simulink model "V2x_TC_CarBreakdownWarning_cs"  (Simulink 7.6)
settings: Solver=ode5  SolverMode=SingleTasking  StartTime=0.0  StopTime=18  FixedStep=1/100  RelTol=1e-3
PreLoadFcn:
  | check_NUTS_defined;
  | 
  | assignin('base',['model_closed_' bdroot],false);addpath('../includes_V2x');
InitFcn:
  | PreScanExperimentInitFcn(bdroot)
StopFcn:
  | PreScanExperimentStopFcn(bdroot)
undefined symbols (not defined in the file or in its folder): acceleration, actorID, actorType, DiscIntNeverNeededParam, GPS_alt, GPS_lat, GPS_long, intmax, lightBarInUse, messageID, Newton, publicActorType, Raphson, rotZ, sigbuilder_block, sireneInUse, trafficLightPriority, turnAdvice, velocity, x_ini_VRML, y_ini_VRML, yawRate, z_ini_VRML
libraries: simulink x61, PreScanSimulinkLibrary x19, PreScanUsefulBlocks x7, simulink_extras x1
(part 5 of 10)

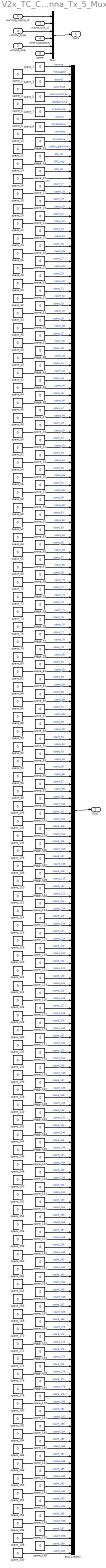
== system V2x_TC_CarBreakdownWarning_cs/BMW_X5_1/Antenna_Tx_5_Mux ==
  warning_signal_id : Inport  SampleTime=TimeStep
  maneuvre_id : Inport  Port=2  SampleTime=TimeStep
  vehicle_type : Inport  Port=3  SampleTime=TimeStep
  brakingcapacity : Inport  Port=4  SampleTime=TimeStep
  vehicle_size : Inport  Port=5  SampleTime=TimeStep
  spare : Inport  Port=6  SampleTime=TimeStep
  Bus Creator : BusCreator  Inputs=200
  Mux : Mux  Inputs=6
  spare_{1..200} (200 alike) : Constant  Value=0  SampleTime=TimeStep
  Out1 : Outport
  Out2 : Outport  Port=2  SampleTime=TimeStep
  wires:
  spare_200/1 -> Bus Creator/200  "spare_200"
  spare_199/1 -> Bus Creator/199  "spare_199"
  spare_198/1 -> Bus Creator/198  "spare_198"
  spare_197/1 -> Bus Creator/197  "spare_197"
  spare_196/1 -> Bus Creator/196  "spare_196"
  spare_195/1 -> Bus Creator/195  "spare_195"
  spare_194/1 -> Bus Creator/194  "spare_194"
  spare_193/1 -> Bus Creator/193  "spare_193"
  spare_192/1 -> Bus Creator/192  "spare_192"
  spare_191/1 -> Bus Creator/191  "spare_191"
  spare_190/1 -> Bus Creator/190  "spare_190"
  spare_189/1 -> Bus Creator/189  "spare_189"
  spare_188/1 -> Bus Creator/188  "spare_188"
  spare_187/1 -> Bus Creator/187  "spare_187"
  spare_186/1 -> Bus Creator/186  "spare_186"
  spare_185/1 -> Bus Creator/185  "spare_185"
  spare_184/1 -> Bus Creator/184  "spare_184"
  spare_183/1 -> Bus Creator/183  "spare_183"
  spare_182/1 -> Bus Creator/182  "spare_182"
  spare_181/1 -> Bus Creator/181  "spare_181"
  spare_180/1 -> Bus Creator/180  "spare_180"
  spare_179/1 -> Bus Creator/179  "spare_179"
  spare_178/1 -> Bus Creator/178  "spare_178"
  spare_177/1 -> Bus Creator/177  "spare_177"
  spare_176/1 -> Bus Creator/176  "spare_176"
  spare_175/1 -> Bus Creator/175  "spare_175"
  spare_174/1 -> Bus Creator/174  "spare_174"
  spare_173/1 -> Bus Creator/173  "spare_173"
  spare_172/1 -> Bus Creator/172  "spare_172"
  spare_171/1 -> Bus Creator/171  "spare_171"
  spare_170/1 -> Bus Creator/170  "spare_170"
  spare_169/1 -> Bus Creator/169  "spare_169"
  spare_168/1 -> Bus Creator/168  "spare_168"
  spare_167/1 -> Bus Creator/167  "spare_167"
  spare_166/1 -> Bus Creator/166  "spare_166"
  spare_165/1 -> Bus Creator/165  "spare_165"
  spare_164/1 -> Bus Creator/164  "spare_164"
  spare_163/1 -> Bus Creator/163  "spare_163"
  spare_162/1 -> Bus Creator/162  "spare_162"
  spare_161/1 -> Bus Creator/161  "spare_161"
  spare_160/1 -> Bus Creator/160  "spare_160"
  spare_159/1 -> Bus Creator/159  "spare_159"
  spare_158/1 -> Bus Creator/158  "spare_158"
  spare_157/1 -> Bus Creator/157  "spare_157"
  spare_156/1 -> Bus Creator/156  "spare_156"
  spare_155/1 -> Bus Creator/155  "spare_155"
  spare_154/1 -> Bus Creator/154  "spare_154"
  spare_153/1 -> Bus Creator/153  "spare_153"
  spare_152/1 -> Bus Creator/152  "spare_152"
  spare_151/1 -> Bus Creator/151  "spare_151"
  spare_150/1 -> Bus Creator/150  "spare_150"
  spare_149/1 -> Bus Creator/149  "spare_149"
  spare_148/1 -> Bus Creator/148  "spare_148"
  spare_147/1 -> Bus Creator/147  "spare_147"
  spare_146/1 -> Bus Creator/146  "spare_146"
  spare_145/1 -> Bus Creator/145  "spare_145"
  spare_144/1 -> Bus Creator/144  "spare_144"
  spare_143/1 -> Bus Creator/143  "spare_143"
  spare_142/1 -> Bus Creator/142  "spare_142"
  spare_141/1 -> Bus Creator/141  "spare_141"
  spare_140/1 -> Bus Creator/140  "spare_140"
  spare_139/1 -> Bus Creator/139  "spare_139"
  spare_138/1 -> Bus Creator/138  "spare_138"
  spare_137/1 -> Bus Creator/137  "spare_137"
  spare_136/1 -> Bus Creator/136  "spare_136"
  spare_135/1 -> Bus Creator/135  "spare_135"
  spare_134/1 -> Bus Creator/134  "spare_134"
  spare_133/1 -> Bus Creator/133  "spare_133"
  spare_132/1 -> Bus Creator/132  "spare_132"
  spare_131/1 -> Bus Creator/131  "spare_131"
  spare_130/1 -> Bus Creator/130  "spare_130"
  spare_129/1 -> Bus Creator/129  "spare_129"
  spare_128/1 -> Bus Creator/128  "spare_128"
  spare_127/1 -> Bus Creator/127  "spare_127"
  spare_126/1 -> Bus Creator/126  "spare_126"
  spare_125/1 -> Bus Creator/125  "spare_125"
  spare_124/1 -> Bus Creator/124  "spare_124"
  spare_123/1 -> Bus Creator/123  "spare_123"
  spare_122/1 -> Bus Creator/122  "spare_122"
  spare_121/1 -> Bus Creator/121  "spare_121"
  spare_120/1 -> Bus Creator/120  "spare_120"
  spare_119/1 -> Bus Creator/119  "spare_119"
  spare_118/1 -> Bus Creator/118  "spare_118"
  spare_117/1 -> Bus Creator/117  "spare_117"
  spare_116/1 -> Bus Creator/116  "spare_116"
  spare_115/1 -> Bus Creator/115  "spare_115"
  spare_114/1 -> Bus Creator/114  "spare_114"
  spare_113/1 -> Bus Creator/113  "spare_113"
  spare_112/1 -> Bus Creator/112  "spare_112"
  spare_111/1 -> Bus Creator/111  "spare_111"
  spare_110/1 -> Bus Creator/110  "spare_110"
  spare_109/1 -> Bus Creator/109  "spare_109"
  spare_108/1 -> Bus Creator/108  "spare_108"
  spare_107/1 -> Bus Creator/107  "spare_107"
  spare_106/1 -> Bus Creator/106  "spare_106"
  spare_105/1 -> Bus Creator/105  "spare_105"
  spare_104/1 -> Bus Creator/104  "spare_104"
  spare_103/1 -> Bus Creator/103  "spare_103"
  spare_102/1 -> Bus Creator/102  "spare_102"
  spare_101/1 -> Bus Creator/101  "spare_101"
  spare_100/1 -> Bus Creator/100  "spare_100"
  spare_99/1 -> Bus Creator/99  "spare_99"
  spare_98/1 -> Bus Creator/98  "spare_98"
  spare_97/1 -> Bus Creator/97  "spare_97"
  spare_96/1 -> Bus Creator/96  "spare_96"
  spare_95/1 -> Bus Creator/95  "spare_95"
  spare_94/1 -> Bus Creator/94  "spare_94"
  spare_93/1 -> Bus Creator/93  "spare_93"
  spare_92/1 -> Bus Creator/92  "spare_92"
  spare_91/1 -> Bus Creator/91  "spare_91"
  spare_90/1 -> Bus Creator/90  "spare_90"
  spare_89/1 -> Bus Creator/89  "spare_89"
  spare_88/1 -> Bus Creator/88  "spare_88"
  spare_87/1 -> Bus Creator/87  "spare_87"
  spare_86/1 -> Bus Creator/86  "spare_86"
  spare_85/1 -> Bus Creator/85  "spare_85"
  spare_84/1 -> Bus Creator/84  "spare_84"
  spare_83/1 -> Bus Creator/83  "spare_83"
  spare_82/1 -> Bus Creator/82  "spare_82"
  spare_81/1 -> Bus Creator/81  "spare_81"
  spare_80/1 -> Bus Creator/80  "spare_80"
  spare_79/1 -> Bus Creator/79  "spare_79"
  spare_78/1 -> Bus Creator/78  "spare_78"
  spare_77/1 -> Bus Creator/77  "spare_77"
  spare_76/1 -> Bus Creator/76  "spare_76"
  spare_75/1 -> Bus Creator/75  "spare_75"
  spare_74/1 -> Bus Creator/74  "spare_74"
  spare_73/1 -> Bus Creator/73  "spare_73"
  spare_72/1 -> Bus Creator/72  "spare_72"
  spare_71/1 -> Bus Creator/71  "spare_71"
  spare_70/1 -> Bus Creator/70  "spare_70"
  spare_69/1 -> Bus Creator/69  "spare_69"
  spare_68/1 -> Bus Creator/68  "spare_68"
  spare_67/1 -> Bus Creator/67  "spare_67"
  spare_66/1 -> Bus Creator/66  "spare_66"
  spare_65/1 -> Bus Creator/65  "spare_65"
  spare_64/1 -> Bus Creator/64  "spare_64"
  spare_63/1 -> Bus Creator/63  "spare_63"
  spare_62/1 -> Bus Creator/62  "spare_62"
  spare_61/1 -> Bus Creator/61  "spare_61"
  spare_60/1 -> Bus Creator/60  "spare_60"
  spare_59/1 -> Bus Creator/59  "spare_59"
  spare_58/1 -> Bus Creator/58  "spare_58"
  spare_57/1 -> Bus Creator/57  "spare_57"
  spare_56/1 -> Bus Creator/56  "spare_56"
  spare_55/1 -> Bus Creator/55  "spare_55"
  spare_54/1 -> Bus Creator/54  "spare_54"
  spare_53/1 -> Bus Creator/53  "spare_53"
  spare_52/1 -> Bus Creator/52  "spare_52"
  spare_51/1 -> Bus Creator/51  "spare_51"
  spare_50/1 -> Bus Creator/50  "spare_50"
  spare_49/1 -> Bus Creator/49  "spare_49"
  spare_48/1 -> Bus Creator/48  "spare_48"
  spare_47/1 -> Bus Creator/47  "spare_47"
  spare_46/1 -> Bus Creator/46  "spare_46"
  spare_45/1 -> Bus Creator/45  "spare_45"
  spare_44/1 -> Bus Creator/44  "spare_44"
  spare_43/1 -> Bus Creator/43  "spare_43"
  spare_42/1 -> Bus Creator/42  "spare_42"
  spare_41/1 -> Bus Creator/41  "spare_41"
  spare_40/1 -> Bus Creator/40  "spare_40"
  spare_39/1 -> Bus Creator/39  "spare_39"
  spare_38/1 -> Bus Creator/38  "spare_38"
  spare_37/1 -> Bus Creator/37  "spare_37"
  spare_36/1 -> Bus Creator/36  "spare_36"
  spare_35/1 -> Bus Creator/35  "spare_35"
  spare_34/1 -> Bus Creator/34  "spare_34"
  spare_33/1 -> Bus Creator/33  "spare_33"
  spare_32/1 -> Bus Creator/32  "spare_32"
  spare_31/1 -> Bus Creator/31  "spare_31"
  spare_30/1 -> Bus Creator/30  "spare_30"
  spare_29/1 -> Bus Creator/29  "spare_29"
  spare_28/1 -> Bus Creator/28  "spare_28"
  spare_27/1 -> Bus Creator/27  "spare_27"
  spare_26/1 -> Bus Creator/26  "spare_26"
  spare_25/1 -> Bus Creator/25  "spare_25"
  spare_24/1 -> Bus Creator/24  "spare_24"
  spare_23/1 -> Bus Creator/23  "spare_23"
  spare_22/1 -> Bus Creator/22  "spare_22"
  spare_21/1 -> Bus Creator/21  "spare_21"
  spare_19/1 -> Bus Creator/19  "spare_19"
  spare_18/1 -> Bus Creator/18  "spare_18"
  spare_17/1 -> Bus Creator/17  "spare_17"
  warning_signal_id/1 -> Mux/1
  maneuvre_id/1 -> Mux/2
  vehicle_type/1 -> Mux/3
  brakingcapacity/1 -> Mux/4
  vehicle_size/1 -> Mux/5
  Mux/1 -> Out1/1
  Bus Creator/1 -> Out2/1
  spare/1 -> Mux/6
  spare_1/1 -> Bus Creator/1  "warning"
  spare_2/1 -> Bus Creator/2  "messageID"
  spare_3/1 -> Bus Creator/3  "actorID"
  spare_4/1 -> Bus Creator/4  "actorType"
  spare_5/1 -> Bus Creator/5  "publicActorType"
  spare_6/1 -> Bus Creator/6  "lightBarInUse"
  spare_7/1 -> Bus Creator/7  "sireneInUse"
  spare_8/1 -> Bus Creator/8  "velocity"
  spare_9/1 -> Bus Creator/9  "acceleration"
  spare_10/1 -> Bus Creator/10  "yawRate"
  spare_11/1 -> Bus Creator/11  "turnAdvice"
  spare_12/1 -> Bus Creator/12  "trafficLightPriority"
  spare_13/1 -> Bus Creator/13  "GPS_lat"
  spare_14/1 -> Bus Creator/14  "GPS_long"
  spare_15/1 -> Bus Creator/15  "GPS_alt"
  spare_16/1 -> Bus Creator/16  "rotZ"
  spare_20/1 -> Bus Creator/20  "spare_20"

== system V2x_TC_CarBreakdownWarning_cs/BMW_X5_1/SELF_Demux ==
  SELF : Inport
  Demux1 : Demux  Outputs=3
  Demux2 : Demux  Outputs=3
  Demux3 : Demux  Outputs=[3 3 1 1]
  Demux4 : Demux  Outputs=3
  Gain : Gain  Gain=180/pi
  Gain1 : Gain  Gain=180/pi
  Selector : Selector  InputPortWidth=3  IndexOptions=Index vector (dialog)  Indices=[3]  OutputSizes=1
  compas converter : Subsystem
  xyz2GPS : PreScanUsefulBlocks/xyz2GPS  CoordinateCount=1  GPS_base=[0.000000 0.000000 0.000]
  x [m] : Outport
  y [m] : Outport  Port=2
  z [m] : Outport  Port=3
  rotx [deg] : Outport  Port=4
  roty [deg] : Outport  Port=5
  rotz [deg] : Outport  Port=6
  GPS lat [deg] : Outport  Port=7
  GPS long [deg] : Outport  Port=8
  GPS alt [m] : Outport  Port=9
  velocity [m/s] : Outport  Port=10
  heading [deg] : Outport  Port=11
  yaw rate [deg/s] : Outport  Port=12
  wires:
  Demux3/4 -> Gain1/1
  Gain1/1 -> yaw rate [deg/s]/1
  Demux3/3 -> velocity [m/s]/1
  compas converter/1(heading [deg]) -> heading [deg]/1
  xyz2GPS/1 -> Demux4/1
  Demux4/3 -> GPS alt [m]/1
  Demux4/2 -> GPS long [deg]/1
  Demux4/1 -> GPS lat [deg]/1
  Demux3/2 -> Gain/1, Selector/1
  Demux3/1 -> xyz2GPS/1, Demux1/1
  SELF/1 -> Demux3/1
  Demux2/3 -> rotz [deg]/1
  Demux2/2 -> roty [deg]/1
  Demux2/1 -> rotx [deg]/1
  Demux1/3 -> z [m]/1
  Demux1/2 -> y [m]/1
  Demux1/1 -> x [m]/1
  Gain/1 -> Demux2/1
  Selector/1 -> compas converter/1(rotz [rad])

== system V2x_TC_CarBreakdownWarning_cs/BMW_X5_1/Trajectories ==
  Traj2State1 : Subsystem  Tag=Traj2State
      settings: DeleteFcn=PreScanBlockDeleteFcn;
      mask Type: PreScan Demux Block:
  Trajectory_4 : Subsystem  Tag=Trajectory  mask(PreScan Source Block: Trajectory){FileName='Trajectory_4.mat', TimeStep=1/100}
      mask prompts: TimeStep "Time Step [s]"
      mask help:
      | The Trajectory block contains the trajectories defined in the PreScan Experiment Editor. The output of the trajectory block is the (vehicle) State.
      |
      | For more information, please click Help.
      mask init: same as V2x_TC_CarBreakdownWarning_cs/Audi_A8_1/Trajectories/Trajectory_1
      settings: DeleteFcn=PreScanBlockDeleteFcn;
      mask Help: eval('openHelp(312)')
      mask Display: fprintf(FileName)
  Trajectory_4_Offset : Constant  Tag=TrajectoryOffset  Value="[0  0  0  0  0  0]"
  State : Outport  Tag=TrajOutport
  wires:
  Trajectory_4/1(trajectory) -> Traj2State1/1(Traj Org)
  Trajectory_4_Offset/1 -> Traj2State1/2(Offset)
  Traj2State1/1(state) -> State/1

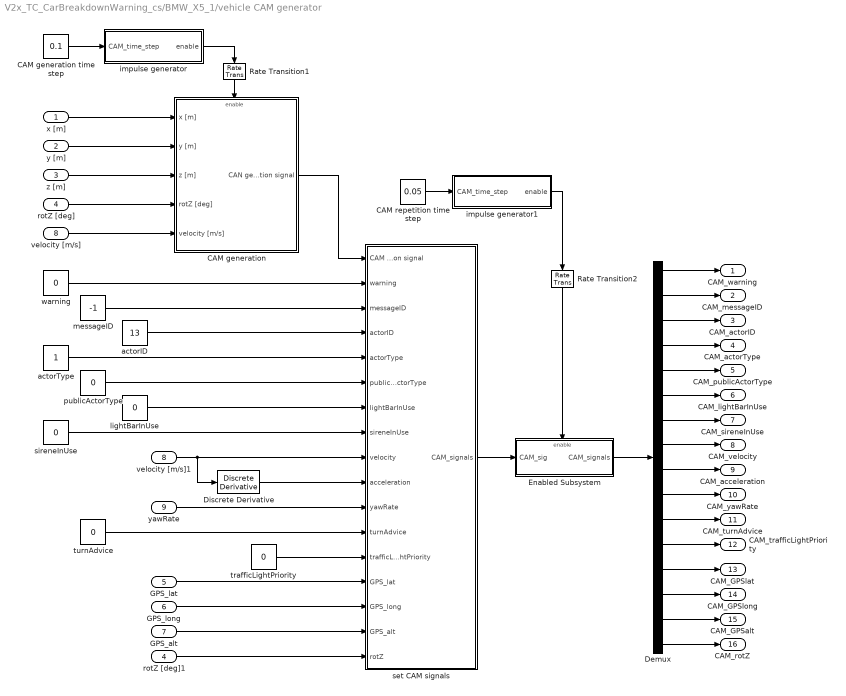
== system V2x_TC_CarBreakdownWarning_cs/BMW_X5_1/vehicle CAM generator ==
  x [m] : Inport
  y [m] : Inport  Port=2
  z [m] : Inport  Port=3
  rotZ [deg] : Inport  Port=4
  GPS_lat : Inport  Port=5
  GPS_long : Inport  Port=6
  GPS_alt : Inport  Port=7
  velocity [m/s] : Inport  Port=8
  yawRate : Inport  Port=9
  CAM generation : Subsystem  TreatAsAtomicUnit=on
  CAM generation time step : Constant  Value=0.1
  CAM repetition time step : Constant  Value=0.05
  Demux : Demux  Outputs=16
  Discrete Derivative : simulink/Discrete/Discrete Derivative  SystemSampleTime=-1  gainval=1.0  ICPrevScaledInput=0.0  OutMin=[]  OutMax=[]  OutDataType=fixdt(1, 16)  OutScaling=2^-10  DoSatur=off
  Enabled Subsystem : Subsystem  TreatAsAtomicUnit=on
  Rate Transition1 : RateTransition  Integrity=off  OutPortSampleTimeOpt=Inherit
  Rate Transition2 : RateTransition  Integrity=off  OutPortSampleTimeOpt=Inherit
  actorID : Constant  Value=13
  actorType : Constant
  impulse generator : Subsystem
  impulse generator1 : Subsystem
  lightBarInUse : Constant  Value=0
  messageID : Constant  Value=-1
  publicActorType : Constant  Value=0
  rotZ [deg]1 : InportShadow  Port=4
  set CAM signals : Subsystem
  sireneInUse : Constant  Value=0
  trafficLightPriority : Constant  Value=0
  turnAdvice : Constant  Value=0
  velocity [m/s]1 : InportShadow  Port=8
  warning : Constant  Value=0
  CAM_warning : Outport
  CAM_messageID : Outport  Port=2
  CAM_actorID : Outport  Port=3
  CAM_actorType : Outport  Port=4
  CAM_publicActorType : Outport  Port=5
  CAM_lightBarInUse : Outport  Port=6
  CAM_sireneInUse : Outport  Port=7
  CAM_velocity : Outport  Port=8
  CAM_acceleration : Outport  Port=9
  CAM_yawRate : Outport  Port=10
  CAM_turnAdvice : Outport  Port=11
  CAM_trafficLightPriority : Outport  Port=12
  CAM_GPSlat : Outport  Port=13
  CAM_GPSlong : Outport  Port=14
  CAM_GPSalt : Outport  Port=15
  CAM_rotZ : Outport  Port=16
  wires:
  CAM generation time step/1 -> impulse generator/1(CAM_time_step)
  CAM repetition time step/1 -> impulse generator1/1(CAM_time_step)
  impulse generator1/1(enable) -> Rate Transition2/1
  warning/1 -> set CAM signals/2(warning)
  messageID/1 -> set CAM signals/3(messageID)
  actorID/1 -> set CAM signals/4(actorID)
  actorType/1 -> set CAM signals/5(actorType)
  publicActorType/1 -> set CAM signals/6(publicActorType)
  lightBarInUse/1 -> set CAM signals/7(lightBarInUse)
  sireneInUse/1 -> set CAM signals/8(sireneInUse)
  velocity [m/s]1/1 -> Discrete Derivative/1, set CAM signals/9(velocity)
  Discrete Derivative/1 -> set CAM signals/10(acceleration)
  yawRate/1 -> set CAM signals/11(yawRate)
  turnAdvice/1 -> set CAM signals/12(turnAdvice)
  trafficLightPriority/1 -> set CAM signals/13(trafficLightPriority)
  GPS_lat/1 -> set CAM signals/14(GPS_lat)
  GPS_long/1 -> set CAM signals/15(GPS_long)
  GPS_alt/1 -> set CAM signals/16(GPS_alt)
  rotZ [deg]1/1 -> set CAM signals/17(rotZ)
  CAM generation/1(CAN generation signal) -> set CAM signals/1(CAM generation signal)
  x [m]/1 -> CAM generation/1(x [m])
  y [m]/1 -> CAM generation/2(y [m])
  z [m]/1 -> CAM generation/3(z [m])
  rotZ [deg]/1 -> CAM generation/4(rotZ [deg])
  velocity [m/s]/1 -> CAM generation/5(velocity [m/s])
  impulse generator/1(enable) -> Rate Transition1/1
  Rate Transition1/1 -> CAM generation/Enable
  set CAM signals/1(CAM_signals) -> Enabled Subsystem/1(CAM_sig)
  Rate Transition2/1 -> Enabled Subsystem/Enable
  Enabled Subsystem/1(CAM_signals) -> Demux/1
  Demux/1 -> CAM_warning/1
  Demux/2 -> CAM_messageID/1
  Demux/3 -> CAM_actorID/1
  Demux/4 -> CAM_actorType/1
  Demux/5 -> CAM_publicActorType/1
  Demux/6 -> CAM_lightBarInUse/1
  Demux/7 -> CAM_sireneInUse/1
  Demux/8 -> CAM_velocity/1
  Demux/9 -> CAM_acceleration/1
  Demux/10 -> CAM_yawRate/1
  Demux/11 -> CAM_turnAdvice/1
  Demux/12 -> CAM_trafficLightPriority/1
  Demux/13 -> CAM_GPSlat/1
  Demux/14 -> CAM_GPSlong/1
  Demux/15 -> CAM_GPSalt/1
  Demux/16 -> CAM_rotZ/1

== system V2x_TC_CarBreakdownWarning_cs/CameraTrolley/Dynamics_Empty ==
  note: For state mode 'Dynamic' positions
      | are not taken into account, as they
      | are computed by integrating velocity.
      | Click annotation for Help.
  Ground_{1..9} (9 alike) : Ground
  MuxState : Subsystem  Tag=MuxState  mask{positioningmode=on, TimeStep=1/100}
      mask prompts: positioningmode "Positioning Mode"; TimeStep "Auto Assigned: Time Step [s]"
      settings: DeleteFcn=PreScanBlockDeleteFcn;
  State : Outport  Tag=StateOutport
  wires:
  MuxState/1(state) -> State/1
  Ground_1/1 -> MuxState/1(x [m])
  Ground_2/1 -> MuxState/2(y [m])
  Ground_3/1 -> MuxState/3(z [m])
  Ground_4/1 -> MuxState/4(dx [m/s])
  Ground_5/1 -> MuxState/5(dy [m/s])
  Ground_6/1 -> MuxState/6(dz [m/s])
  Ground_7/1 -> MuxState/7(R [rad])
  Ground_8/1 -> MuxState/8(P [rad])
  Ground_9/1 -> MuxState/9(Y [rad])

== system V2x_TC_CarBreakdownWarning_cs/CameraTrolley/SELF_Demux ==
  SELF : Inport
  Demux1 : Demux  Outputs=3
  Demux2 : Demux  Outputs=3
  Demux3 : Demux  Outputs=[3 3 1 1]
  Demux4 : Demux  Outputs=3
  Gain : Gain  Gain=180/pi
  Gain1 : Gain  Gain=180/pi
  Selector : Selector  InputPortWidth=3  IndexOptions=Index vector (dialog)  Indices=[3]  OutputSizes=1
  compas converter : Subsystem
  xyz2GPS : PreScanUsefulBlocks/xyz2GPS  CoordinateCount=1  GPS_base=[0.000000 0.000000 0.000]
  x [m] : Outport
  y [m] : Outport  Port=2
  z [m] : Outport  Port=3
  rotx [deg] : Outport  Port=4
  roty [deg] : Outport  Port=5
  rotz [deg] : Outport  Port=6
  GPS lat [deg] : Outport  Port=7
  GPS long [deg] : Outport  Port=8
  GPS alt [m] : Outport  Port=9
  velocity [m/s] : Outport  Port=10
  heading [deg] : Outport  Port=11
  yaw rate [deg/s] : Outport  Port=12
  wires:
  Demux3/4 -> Gain1/1
  Gain1/1 -> yaw rate [deg/s]/1
  Demux3/3 -> velocity [m/s]/1
  compas converter/1(heading [deg]) -> heading [deg]/1
  xyz2GPS/1 -> Demux4/1
  Demux4/3 -> GPS alt [m]/1
  Demux4/2 -> GPS long [deg]/1
  Demux4/1 -> GPS lat [deg]/1
  Demux3/2 -> Gain/1, Selector/1
  Demux3/1 -> xyz2GPS/1, Demux1/1
  SELF/1 -> Demux3/1
  Demux2/3 -> rotz [deg]/1
  Demux2/2 -> roty [deg]/1
  Demux2/1 -> rotx [deg]/1
  Demux1/3 -> z [m]/1
  Demux1/2 -> y [m]/1
  Demux1/1 -> x [m]/1
  Gain/1 -> Demux2/1
  Selector/1 -> compas converter/1(rotz [rad])

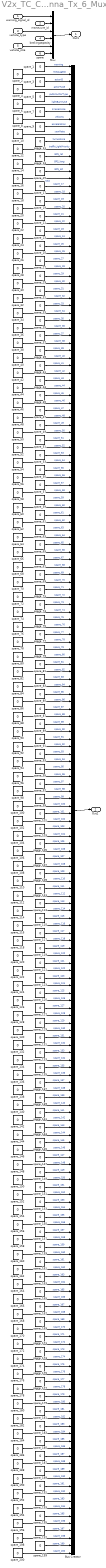
== system V2x_TC_CarBreakdownWarning_cs/Fiat_Bravo_1/Antenna_Tx_6_Mux ==
  warning_signal_id : Inport  SampleTime=TimeStep
  maneuvre_id : Inport  Port=2  SampleTime=TimeStep
  vehicle_type : Inport  Port=3  SampleTime=TimeStep
  brakingcapacity : Inport  Port=4  SampleTime=TimeStep
  vehicle_size : Inport  Port=5  SampleTime=TimeStep
  spare : Inport  Port=6  SampleTime=TimeStep
  Bus Creator : BusCreator  Inputs=200
  Mux : Mux  Inputs=6
  spare_{1..200} (200 alike) : Constant  Value=0  SampleTime=TimeStep
  Out1 : Outport
  Out2 : Outport  Port=2  SampleTime=TimeStep
  wires:
  spare_200/1 -> Bus Creator/200  "spare_200"
  spare_199/1 -> Bus Creator/199  "spare_199"
  spare_198/1 -> Bus Creator/198  "spare_198"
  spare_197/1 -> Bus Creator/197  "spare_197"
  spare_196/1 -> Bus Creator/196  "spare_196"
  spare_195/1 -> Bus Creator/195  "spare_195"
  spare_194/1 -> Bus Creator/194  "spare_194"
  spare_193/1 -> Bus Creator/193  "spare_193"
  spare_192/1 -> Bus Creator/192  "spare_192"
  spare_191/1 -> Bus Creator/191  "spare_191"
  spare_190/1 -> Bus Creator/190  "spare_190"
  spare_189/1 -> Bus Creator/189  "spare_189"
  spare_188/1 -> Bus Creator/188  "spare_188"
  spare_187/1 -> Bus Creator/187  "spare_187"
  spare_186/1 -> Bus Creator/186  "spare_186"
  spare_185/1 -> Bus Creator/185  "spare_185"
  spare_184/1 -> Bus Creator/184  "spare_184"
  spare_183/1 -> Bus Creator/183  "spare_183"
  spare_182/1 -> Bus Creator/182  "spare_182"
  spare_181/1 -> Bus Creator/181  "spare_181"
  spare_180/1 -> Bus Creator/180  "spare_180"
  spare_179/1 -> Bus Creator/179  "spare_179"
  spare_178/1 -> Bus Creator/178  "spare_178"
  spare_177/1 -> Bus Creator/177  "spare_177"
  spare_176/1 -> Bus Creator/176  "spare_176"
  spare_175/1 -> Bus Creator/175  "spare_175"
  spare_174/1 -> Bus Creator/174  "spare_174"
  spare_173/1 -> Bus Creator/173  "spare_173"
  spare_172/1 -> Bus Creator/172  "spare_172"
  spare_171/1 -> Bus Creator/171  "spare_171"
  spare_170/1 -> Bus Creator/170  "spare_170"
  spare_169/1 -> Bus Creator/169  "spare_169"
  spare_168/1 -> Bus Creator/168  "spare_168"
  spare_167/1 -> Bus Creator/167  "spare_167"
  spare_166/1 -> Bus Creator/166  "spare_166"
  spare_165/1 -> Bus Creator/165  "spare_165"
  spare_164/1 -> Bus Creator/164  "spare_164"
  spare_163/1 -> Bus Creator/163  "spare_163"
  spare_162/1 -> Bus Creator/162  "spare_162"
  spare_161/1 -> Bus Creator/161  "spare_161"
  spare_160/1 -> Bus Creator/160  "spare_160"
  spare_159/1 -> Bus Creator/159  "spare_159"
  spare_158/1 -> Bus Creator/158  "spare_158"
  spare_157/1 -> Bus Creator/157  "spare_157"
  spare_156/1 -> Bus Creator/156  "spare_156"
  spare_155/1 -> Bus Creator/155  "spare_155"
  spare_154/1 -> Bus Creator/154  "spare_154"
  spare_153/1 -> Bus Creator/153  "spare_153"
  spare_152/1 -> Bus Creator/152  "spare_152"
  spare_151/1 -> Bus Creator/151  "spare_151"
  spare_150/1 -> Bus Creator/150  "spare_150"
  spare_149/1 -> Bus Creator/149  "spare_149"
  spare_148/1 -> Bus Creator/148  "spare_148"
  spare_147/1 -> Bus Creator/147  "spare_147"
  spare_146/1 -> Bus Creator/146  "spare_146"
  spare_145/1 -> Bus Creator/145  "spare_145"
  spare_144/1 -> Bus Creator/144  "spare_144"
  spare_143/1 -> Bus Creator/143  "spare_143"
  spare_142/1 -> Bus Creator/142  "spare_142"
  spare_141/1 -> Bus Creator/141  "spare_141"
  spare_140/1 -> Bus Creator/140  "spare_140"
  spare_139/1 -> Bus Creator/139  "spare_139"
  spare_138/1 -> Bus Creator/138  "spare_138"
  spare_137/1 -> Bus Creator/137  "spare_137"
  spare_136/1 -> Bus Creator/136  "spare_136"
  spare_135/1 -> Bus Creator/135  "spare_135"
  spare_134/1 -> Bus Creator/134  "spare_134"
  spare_133/1 -> Bus Creator/133  "spare_133"
  spare_132/1 -> Bus Creator/132  "spare_132"
  spare_131/1 -> Bus Creator/131  "spare_131"
  spare_130/1 -> Bus Creator/130  "spare_130"
  spare_129/1 -> Bus Creator/129  "spare_129"
  spare_128/1 -> Bus Creator/128  "spare_128"
  spare_127/1 -> Bus Creator/127  "spare_127"
  spare_126/1 -> Bus Creator/126  "spare_126"
  spare_125/1 -> Bus Creator/125  "spare_125"
  spare_124/1 -> Bus Creator/124  "spare_124"
  spare_123/1 -> Bus Creator/123  "spare_123"
  spare_122/1 -> Bus Creator/122  "spare_122"
  spare_121/1 -> Bus Creator/121  "spare_121"
  spare_120/1 -> Bus Creator/120  "spare_120"
  spare_119/1 -> Bus Creator/119  "spare_119"
  spare_118/1 -> Bus Creator/118  "spare_118"
  spare_117/1 -> Bus Creator/117  "spare_117"
  spare_116/1 -> Bus Creator/116  "spare_116"
  spare_115/1 -> Bus Creator/115  "spare_115"
  spare_114/1 -> Bus Creator/114  "spare_114"
  spare_113/1 -> Bus Creator/113  "spare_113"
  spare_112/1 -> Bus Creator/112  "spare_112"
  spare_111/1 -> Bus Creator/111  "spare_111"
  spare_110/1 -> Bus Creator/110  "spare_110"
  spare_109/1 -> Bus Creator/109  "spare_109"
  spare_108/1 -> Bus Creator/108  "spare_108"
  spare_107/1 -> Bus Creator/107  "spare_107"
  spare_106/1 -> Bus Creator/106  "spare_106"
  spare_105/1 -> Bus Creator/105  "spare_105"
  spare_104/1 -> Bus Creator/104  "spare_104"
  spare_103/1 -> Bus Creator/103  "spare_103"
  spare_102/1 -> Bus Creator/102  "spare_102"
  spare_101/1 -> Bus Creator/101  "spare_101"
  spare_100/1 -> Bus Creator/100  "spare_100"
  spare_99/1 -> Bus Creator/99  "spare_99"
  spare_98/1 -> Bus Creator/98  "spare_98"
  spare_97/1 -> Bus Creator/97  "spare_97"
  spare_96/1 -> Bus Creator/96  "spare_96"
  spare_95/1 -> Bus Creator/95  "spare_95"
  spare_94/1 -> Bus Creator/94  "spare_94"
  spare_93/1 -> Bus Creator/93  "spare_93"
  spare_92/1 -> Bus Creator/92  "spare_92"
  spare_91/1 -> Bus Creator/91  "spare_91"
  spare_90/1 -> Bus Creator/90  "spare_90"
  spare_89/1 -> Bus Creator/89  "spare_89"
  spare_88/1 -> Bus Creator/88  "spare_88"
  spare_87/1 -> Bus Creator/87  "spare_87"
  spare_86/1 -> Bus Creator/86  "spare_86"
  spare_85/1 -> Bus Creator/85  "spare_85"
  spare_84/1 -> Bus Creator/84  "spare_84"
  spare_83/1 -> Bus Creator/83  "spare_83"
  spare_82/1 -> Bus Creator/82  "spare_82"
  spare_81/1 -> Bus Creator/81  "spare_81"
  spare_80/1 -> Bus Creator/80  "spare_80"
  spare_79/1 -> Bus Creator/79  "spare_79"
  spare_78/1 -> Bus Creator/78  "spare_78"
  spare_77/1 -> Bus Creator/77  "spare_77"
  spare_76/1 -> Bus Creator/76  "spare_76"
  spare_75/1 -> Bus Creator/75  "spare_75"
  spare_74/1 -> Bus Creator/74  "spare_74"
  spare_73/1 -> Bus Creator/73  "spare_73"
  spare_72/1 -> Bus Creator/72  "spare_72"
  spare_71/1 -> Bus Creator/71  "spare_71"
  spare_70/1 -> Bus Creator/70  "spare_70"
  spare_69/1 -> Bus Creator/69  "spare_69"
  spare_68/1 -> Bus Creator/68  "spare_68"
  spare_67/1 -> Bus Creator/67  "spare_67"
  spare_66/1 -> Bus Creator/66  "spare_66"
  spare_65/1 -> Bus Creator/65  "spare_65"
  spare_64/1 -> Bus Creator/64  "spare_64"
  spare_63/1 -> Bus Creator/63  "spare_63"
  spare_62/1 -> Bus Creator/62  "spare_62"
  spare_61/1 -> Bus Creator/61  "spare_61"
  spare_60/1 -> Bus Creator/60  "spare_60"
  spare_59/1 -> Bus Creator/59  "spare_59"
  spare_58/1 -> Bus Creator/58  "spare_58"
  spare_57/1 -> Bus Creator/57  "spare_57"
  spare_56/1 -> Bus Creator/56  "spare_56"
  spare_55/1 -> Bus Creator/55  "spare_55"
  spare_54/1 -> Bus Creator/54  "spare_54"
  spare_53/1 -> Bus Creator/53  "spare_53"
  spare_52/1 -> Bus Creator/52  "spare_52"
  spare_51/1 -> Bus Creator/51  "spare_51"
  spare_50/1 -> Bus Creator/50  "spare_50"
  spare_49/1 -> Bus Creator/49  "spare_49"
  spare_48/1 -> Bus Creator/48  "spare_48"
  spare_47/1 -> Bus Creator/47  "spare_47"
  spare_46/1 -> Bus Creator/46  "spare_46"
  spare_45/1 -> Bus Creator/45  "spare_45"
  spare_44/1 -> Bus Creator/44  "spare_44"
  spare_43/1 -> Bus Creator/43  "spare_43"
  spare_42/1 -> Bus Creator/42  "spare_42"
  spare_41/1 -> Bus Creator/41  "spare_41"
  spare_40/1 -> Bus Creator/40  "spare_40"
  spare_39/1 -> Bus Creator/39  "spare_39"
  spare_38/1 -> Bus Creator/38  "spare_38"
  spare_37/1 -> Bus Creator/37  "spare_37"
  spare_36/1 -> Bus Creator/36  "spare_36"
  spare_35/1 -> Bus Creator/35  "spare_35"
  spare_34/1 -> Bus Creator/34  "spare_34"
  spare_33/1 -> Bus Creator/33  "spare_33"
  spare_32/1 -> Bus Creator/32  "spare_32"
  spare_31/1 -> Bus Creator/31  "spare_31"
  spare_30/1 -> Bus Creator/30  "spare_30"
  spare_29/1 -> Bus Creator/29  "spare_29"
  spare_28/1 -> Bus Creator/28  "spare_28"
  spare_27/1 -> Bus Creator/27  "spare_27"
  spare_26/1 -> Bus Creator/26  "spare_26"
  spare_25/1 -> Bus Creator/25  "spare_25"
  spare_24/1 -> Bus Creator/24  "spare_24"
  spare_23/1 -> Bus Creator/23  "spare_23"
  spare_22/1 -> Bus Creator/22  "spare_22"
  spare_21/1 -> Bus Creator/21  "spare_21"
  spare_19/1 -> Bus Creator/19  "spare_19"
  spare_18/1 -> Bus Creator/18  "spare_18"
  spare_17/1 -> Bus Creator/17  "spare_17"
  warning_signal_id/1 -> Mux/1
  maneuvre_id/1 -> Mux/2
  vehicle_type/1 -> Mux/3
  brakingcapacity/1 -> Mux/4
  vehicle_size/1 -> Mux/5
  Mux/1 -> Out1/1
  Bus Creator/1 -> Out2/1
  spare/1 -> Mux/6
  spare_1/1 -> Bus Creator/1  "warning"
  spare_2/1 -> Bus Creator/2  "messageID"
  spare_3/1 -> Bus Creator/3  "actorID"
  spare_4/1 -> Bus Creator/4  "actorType"
  spare_5/1 -> Bus Creator/5  "publicActorType"
  spare_6/1 -> Bus Creator/6  "lightBarInUse"
  spare_7/1 -> Bus Creator/7  "sireneInUse"
  spare_8/1 -> Bus Creator/8  "velocity"
  spare_9/1 -> Bus Creator/9  "acceleration"
  spare_10/1 -> Bus Creator/10  "yawRate"
  spare_11/1 -> Bus Creator/11  "turnAdvice"
  spare_12/1 -> Bus Creator/12  "trafficLightPriority"
  spare_13/1 -> Bus Creator/13  "GPS_lat"
  spare_14/1 -> Bus Creator/14  "GPS_long"
  spare_15/1 -> Bus Creator/15  "GPS_alt"
  spare_16/1 -> Bus Creator/16  "rotZ"
  spare_20/1 -> Bus Creator/20  "spare_20"

== system V2x_TC_CarBreakdownWarning_cs/Fiat_Bravo_1/SELF_Demux ==
  SELF : Inport
  Demux1 : Demux  Outputs=3
  Demux2 : Demux  Outputs=3
  Demux3 : Demux  Outputs=[3 3 1 1]
  Demux4 : Demux  Outputs=3
  Gain : Gain  Gain=180/pi
  Gain1 : Gain  Gain=180/pi
  Selector : Selector  InputPortWidth=3  IndexOptions=Index vector (dialog)  Indices=[3]  OutputSizes=1
  compas converter : Subsystem
  xyz2GPS : PreScanUsefulBlocks/xyz2GPS  CoordinateCount=1  GPS_base=[0.000000 0.000000 0.000]
  x [m] : Outport
  y [m] : Outport  Port=2
  z [m] : Outport  Port=3
  rotx [deg] : Outport  Port=4
  roty [deg] : Outport  Port=5
  rotz [deg] : Outport  Port=6
  GPS lat [deg] : Outport  Port=7
  GPS long [deg] : Outport  Port=8
  GPS alt [m] : Outport  Port=9
  velocity [m/s] : Outport  Port=10
  heading [deg] : Outport  Port=11
  yaw rate [deg/s] : Outport  Port=12
  wires:
  Demux3/4 -> Gain1/1
  Gain1/1 -> yaw rate [deg/s]/1
  Demux3/3 -> velocity [m/s]/1
  compas converter/1(heading [deg]) -> heading [deg]/1
  xyz2GPS/1 -> Demux4/1
  Demux4/3 -> GPS alt [m]/1
  Demux4/2 -> GPS long [deg]/1
  Demux4/1 -> GPS lat [deg]/1
  Demux3/2 -> Gain/1, Selector/1
  Demux3/1 -> xyz2GPS/1, Demux1/1
  SELF/1 -> Demux3/1
  Demux2/3 -> rotz [deg]/1
  Demux2/2 -> roty [deg]/1
  Demux2/1 -> rotx [deg]/1
  Demux1/3 -> z [m]/1
  Demux1/2 -> y [m]/1
  Demux1/1 -> x [m]/1
  Gain/1 -> Demux2/1
  Selector/1 -> compas converter/1(rotz [rad])

== system V2x_TC_CarBreakdownWarning_cs/Fiat_Bravo_1/Trajectories ==
  Traj2State1 : Subsystem  Tag=Traj2State
      settings: DeleteFcn=PreScanBlockDeleteFcn;
      mask Type: PreScan Demux Block:
  Trajectory_3 : Subsystem  Tag=Trajectory  mask(PreScan Source Block: Trajectory){FileName='Trajectory_3.mat', TimeStep=1/100}
      mask prompts: TimeStep "Time Step [s]"
      mask help:
      | The Trajectory block contains the trajectories defined in the PreScan Experiment Editor. The output of the trajectory block is the (vehicle) State.
      |
      | For more information, please click Help.
      mask init: same as V2x_TC_CarBreakdownWarning_cs/Audi_A8_1/Trajectories/Trajectory_1
      settings: DeleteFcn=PreScanBlockDeleteFcn;
      mask Help: eval('openHelp(312)')
      mask Display: fprintf(FileName)
  Trajectory_3_Offset : Constant  Tag=TrajectoryOffset  Value="[0  0  0  0  0  0]"
  State : Outport  Tag=TrajOutport
  wires:
  Trajectory_3/1(trajectory) -> Traj2State1/1(Traj Org)
  Trajectory_3_Offset/1 -> Traj2State1/2(Offset)
  Traj2State1/1(state) -> State/1

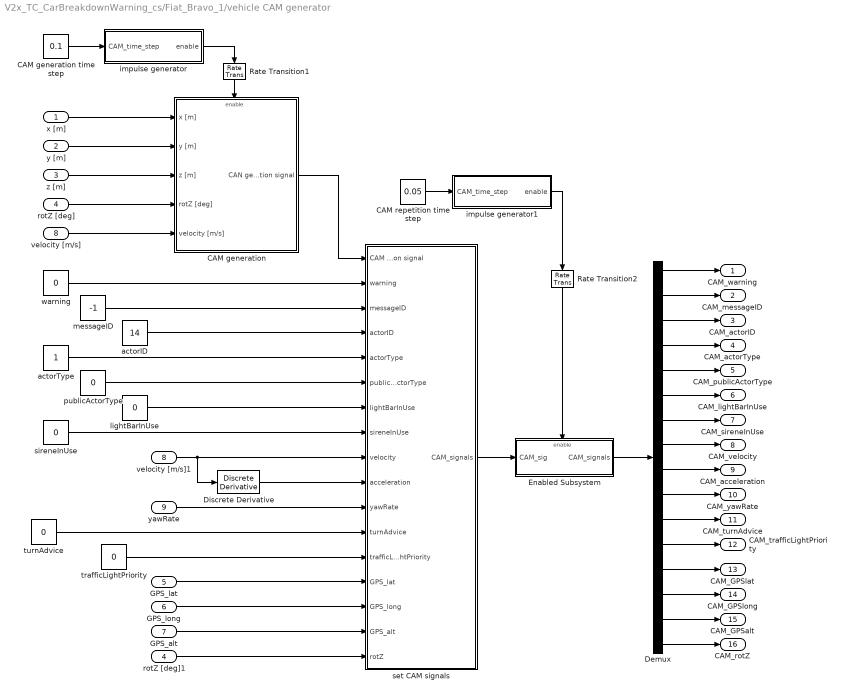
== system V2x_TC_CarBreakdownWarning_cs/Fiat_Bravo_1/vehicle CAM generator ==
  x [m] : Inport
  y [m] : Inport  Port=2
  z [m] : Inport  Port=3
  rotZ [deg] : Inport  Port=4
  GPS_lat : Inport  Port=5
  GPS_long : Inport  Port=6
  GPS_alt : Inport  Port=7
  velocity [m/s] : Inport  Port=8
  yawRate : Inport  Port=9
  CAM generation : Subsystem  TreatAsAtomicUnit=on
  CAM generation time step : Constant  Value=0.1
  CAM repetition time step : Constant  Value=0.05
  Demux : Demux  Outputs=16
  Discrete Derivative : simulink/Discrete/Discrete Derivative  SystemSampleTime=-1  gainval=1.0  ICPrevScaledInput=0.0  OutMin=[]  OutMax=[]  OutDataType=fixdt(1, 16)  OutScaling=2^-10  DoSatur=off
  Enabled Subsystem : Subsystem  TreatAsAtomicUnit=on
  Rate Transition1 : RateTransition  Integrity=off  OutPortSampleTimeOpt=Inherit
  Rate Transition2 : RateTransition  Integrity=off  OutPortSampleTimeOpt=Inherit
  actorID : Constant  Value=14
  actorType : Constant
  impulse generator : Subsystem
  impulse generator1 : Subsystem
  lightBarInUse : Constant  Value=0
  messageID : Constant  Value=-1
  publicActorType : Constant  Value=0
  rotZ [deg]1 : InportShadow  Port=4
  set CAM signals : Subsystem
  sireneInUse : Constant  Value=0
  trafficLightPriority : Constant  Value=0
  turnAdvice : Constant  Value=0
  velocity [m/s]1 : InportShadow  Port=8
  warning : Constant  Value=0
  CAM_warning : Outport
  CAM_messageID : Outport  Port=2
  CAM_actorID : Outport  Port=3
  CAM_actorType : Outport  Port=4
  CAM_publicActorType : Outport  Port=5
  CAM_lightBarInUse : Outport  Port=6
  CAM_sireneInUse : Outport  Port=7
  CAM_velocity : Outport  Port=8
  CAM_acceleration : Outport  Port=9
  CAM_yawRate : Outport  Port=10
  CAM_turnAdvice : Outport  Port=11
  CAM_trafficLightPriority : Outport  Port=12
  CAM_GPSlat : Outport  Port=13
  CAM_GPSlong : Outport  Port=14
  CAM_GPSalt : Outport  Port=15
  CAM_rotZ : Outport  Port=16
  wires:
  CAM generation time step/1 -> impulse generator/1(CAM_time_step)
  CAM repetition time step/1 -> impulse generator1/1(CAM_time_step)
  impulse generator1/1(enable) -> Rate Transition2/1
  warning/1 -> set CAM signals/2(warning)
  messageID/1 -> set CAM signals/3(messageID)
  actorID/1 -> set CAM signals/4(actorID)
  actorType/1 -> set CAM signals/5(actorType)
  publicActorType/1 -> set CAM signals/6(publicActorType)
  lightBarInUse/1 -> set CAM signals/7(lightBarInUse)
  sireneInUse/1 -> set CAM signals/8(sireneInUse)
  velocity [m/s]1/1 -> Discrete Derivative/1, set CAM signals/9(velocity)
  Discrete Derivative/1 -> set CAM signals/10(acceleration)
  yawRate/1 -> set CAM signals/11(yawRate)
  turnAdvice/1 -> set CAM signals/12(turnAdvice)
  trafficLightPriority/1 -> set CAM signals/13(trafficLightPriority)
  GPS_lat/1 -> set CAM signals/14(GPS_lat)
  GPS_long/1 -> set CAM signals/15(GPS_long)
  GPS_alt/1 -> set CAM signals/16(GPS_alt)
  rotZ [deg]1/1 -> set CAM signals/17(rotZ)
  CAM generation/1(CAN generation signal) -> set CAM signals/1(CAM generation signal)
  x [m]/1 -> CAM generation/1(x [m])
  y [m]/1 -> CAM generation/2(y [m])
  z [m]/1 -> CAM generation/3(z [m])
  rotZ [deg]/1 -> CAM generation/4(rotZ [deg])
  velocity [m/s]/1 -> CAM generation/5(velocity [m/s])
  impulse generator/1(enable) -> Rate Transition1/1
  Rate Transition1/1 -> CAM generation/Enable
  set CAM signals/1(CAM_signals) -> Enabled Subsystem/1(CAM_sig)
  Rate Transition2/1 -> Enabled Subsystem/Enable
  Enabled Subsystem/1(CAM_signals) -> Demux/1
  Demux/1 -> CAM_warning/1
  Demux/2 -> CAM_messageID/1
  Demux/3 -> CAM_actorID/1
  Demux/4 -> CAM_actorType/1
  Demux/5 -> CAM_publicActorType/1
  Demux/6 -> CAM_lightBarInUse/1
  Demux/7 -> CAM_sireneInUse/1
  Demux/8 -> CAM_velocity/1
  Demux/9 -> CAM_acceleration/1
  Demux/10 -> CAM_yawRate/1
  Demux/11 -> CAM_turnAdvice/1
  Demux/12 -> CAM_trafficLightPriority/1
  Demux/13 -> CAM_GPSlat/1
  Demux/14 -> CAM_GPSlong/1
  Demux/15 -> CAM_GPSalt/1
  Demux/16 -> CAM_rotZ/1

== system V2x_TC_CarBreakdownWarning_cs/STATE_Audi_A8_1/Acceleration ==
  Y : Inport
  Assignment : Assignment  IndexMode=Zero-based  SampleTime=TimeStep  IndexOptions=Starting index (dialog)  Indices=PortIndex  OutputSizes=[1 1]
  Data Store Read : DataStoreRead  DataStoreName=SimCoreActuators  SampleTime=TimeStep
  Data Store Write : DataStoreWrite  DataStoreName=SimCoreActuators
  wires:
  Assignment/1 -> Data Store Write/1
  Data Store Read/1 -> Assignment/1
  Y/1 -> Assignment/2

== system V2x_TC_CarBreakdownWarning_cs/STATE_Audi_A8_1/Position ==
  Y : Inport
  Assignment : Assignment  IndexMode=Zero-based  SampleTime=TimeStep  IndexOptions=Starting index (dialog)  Indices=PortIndex  OutputSizes=[1 1]
  Data Store Read : DataStoreRead  DataStoreName=SimCoreActuators  SampleTime=TimeStep
  Data Store Write : DataStoreWrite  DataStoreName=SimCoreActuators
  wires:
  Y/1 -> Assignment/2
  Data Store Read/1 -> Assignment/1
  Assignment/1 -> Data Store Write/1

== system V2x_TC_CarBreakdownWarning_cs/STATE_Audi_A8_1/RPY ==
  Y : Inport
  Assignment : Assignment  IndexMode=Zero-based  SampleTime=TimeStep  IndexOptions=Starting index (dialog)  Indices=PortIndex  OutputSizes=[1 1]
  Data Store Read : DataStoreRead  DataStoreName=SimCoreActuators  SampleTime=TimeStep
  Data Store Write : DataStoreWrite  DataStoreName=SimCoreActuators
  wires:
  Assignment/1 -> Data Store Write/1
  Data Store Read/1 -> Assignment/1
  Y/1 -> Assignment/2

== system V2x_TC_CarBreakdownWarning_cs/STATE_Audi_A8_1/Velocity ==
  Y : Inport
  Assignment : Assignment  IndexMode=Zero-based  SampleTime=TimeStep  IndexOptions=Starting index (dialog)  Indices=PortIndex  OutputSizes=[1 1]
  Data Store Read : DataStoreRead  DataStoreName=SimCoreActuators  SampleTime=TimeStep
  Data Store Write : DataStoreWrite  DataStoreName=SimCoreActuators
  wires:
  Assignment/1 -> Data Store Write/1
  Data Store Read/1 -> Assignment/1
  Y/1 -> Assignment/2

== system V2x_TC_CarBreakdownWarning_cs/STATE_Audi_A8_1/velRPY ==
  Y : Inport
  Assignment : Assignment  IndexMode=Zero-based  SampleTime=TimeStep  IndexOptions=Starting index (dialog)  Indices=PortIndex  OutputSizes=[1 1]
  Data Store Read : DataStoreRead  DataStoreName=SimCoreActuators  SampleTime=TimeStep
  Data Store Write : DataStoreWrite  DataStoreName=SimCoreActuators
  wires:
  Assignment/1 -> Data Store Write/1
  Data Store Read/1 -> Assignment/1
  Y/1 -> Assignment/2

== system V2x_TC_CarBreakdownWarning_cs/STATE_BMW_X5_1/Acceleration ==
  Y : Inport
  Assignment : Assignment  IndexMode=Zero-based  SampleTime=TimeStep  IndexOptions=Starting index (dialog)  Indices=PortIndex  OutputSizes=[1 1]
  Data Store Read : DataStoreRead  DataStoreName=SimCoreActuators  SampleTime=TimeStep
  Data Store Write : DataStoreWrite  DataStoreName=SimCoreActuators
  wires:
  Assignment/1 -> Data Store Write/1
  Data Store Read/1 -> Assignment/1
  Y/1 -> Assignment/2

== system V2x_TC_CarBreakdownWarning_cs/STATE_BMW_X5_1/Position ==
  Y : Inport
  Assignment : Assignment  IndexMode=Zero-based  SampleTime=TimeStep  IndexOptions=Starting index (dialog)  Indices=PortIndex  OutputSizes=[1 1]
  Data Store Read : DataStoreRead  DataStoreName=SimCoreActuators  SampleTime=TimeStep
  Data Store Write : DataStoreWrite  DataStoreName=SimCoreActuators
  wires:
  Y/1 -> Assignment/2
  Data Store Read/1 -> Assignment/1
  Assignment/1 -> Data Store Write/1

== system V2x_TC_CarBreakdownWarning_cs/STATE_BMW_X5_1/RPY ==
  Y : Inport
  Assignment : Assignment  IndexMode=Zero-based  SampleTime=TimeStep  IndexOptions=Starting index (dialog)  Indices=PortIndex  OutputSizes=[1 1]
  Data Store Read : DataStoreRead  DataStoreName=SimCoreActuators  SampleTime=TimeStep
  Data Store Write : DataStoreWrite  DataStoreName=SimCoreActuators
  wires:
  Assignment/1 -> Data Store Write/1
  Data Store Read/1 -> Assignment/1
  Y/1 -> Assignment/2

== system V2x_TC_CarBreakdownWarning_cs/STATE_BMW_X5_1/Velocity ==
  Y : Inport
  Assignment : Assignment  IndexMode=Zero-based  SampleTime=TimeStep  IndexOptions=Starting index (dialog)  Indices=PortIndex  OutputSizes=[1 1]
  Data Store Read : DataStoreRead  DataStoreName=SimCoreActuators  SampleTime=TimeStep
  Data Store Write : DataStoreWrite  DataStoreName=SimCoreActuators
  wires:
  Assignment/1 -> Data Store Write/1
  Data Store Read/1 -> Assignment/1
  Y/1 -> Assignment/2

== system V2x_TC_CarBreakdownWarning_cs/STATE_BMW_X5_1/velRPY ==
  Y : Inport
  Assignment : Assignment  IndexMode=Zero-based  SampleTime=TimeStep  IndexOptions=Starting index (dialog)  Indices=PortIndex  OutputSizes=[1 1]
  Data Store Read : DataStoreRead  DataStoreName=SimCoreActuators  SampleTime=TimeStep
  Data Store Write : DataStoreWrite  DataStoreName=SimCoreActuators
  wires:
  Assignment/1 -> Data Store Write/1
  Data Store Read/1 -> Assignment/1
  Y/1 -> Assignment/2

== system V2x_TC_CarBreakdownWarning_cs/STATE_CameraTrolley/Acceleration ==
  Y : Inport
  Assignment : Assignment  IndexMode=Zero-based  SampleTime=TimeStep  IndexOptions=Starting index (dialog)  Indices=PortIndex  OutputSizes=[1 1]
  Data Store Read : DataStoreRead  DataStoreName=SimCoreActuators  SampleTime=TimeStep
  Data Store Write : DataStoreWrite  DataStoreName=SimCoreActuators
  wires:
  Assignment/1 -> Data Store Write/1
  Data Store Read/1 -> Assignment/1
  Y/1 -> Assignment/2

== system V2x_TC_CarBreakdownWarning_cs/STATE_CameraTrolley/Position ==
  Y : Inport
  Assignment : Assignment  IndexMode=Zero-based  SampleTime=TimeStep  IndexOptions=Starting index (dialog)  Indices=PortIndex  OutputSizes=[1 1]
  Data Store Read : DataStoreRead  DataStoreName=SimCoreActuators  SampleTime=TimeStep
  Data Store Write : DataStoreWrite  DataStoreName=SimCoreActuators
  wires:
  Y/1 -> Assignment/2
  Data Store Read/1 -> Assignment/1
  Assignment/1 -> Data Store Write/1

== system V2x_TC_CarBreakdownWarning_cs/STATE_CameraTrolley/RPY ==
  Y : Inport
  Assignment : Assignment  IndexMode=Zero-based  SampleTime=TimeStep  IndexOptions=Starting index (dialog)  Indices=PortIndex  OutputSizes=[1 1]
  Data Store Read : DataStoreRead  DataStoreName=SimCoreActuators  SampleTime=TimeStep
  Data Store Write : DataStoreWrite  DataStoreName=SimCoreActuators
  wires:
  Assignment/1 -> Data Store Write/1
  Data Store Read/1 -> Assignment/1
  Y/1 -> Assignment/2

== system V2x_TC_CarBreakdownWarning_cs/STATE_CameraTrolley/Velocity ==
  Y : Inport
  Assignment : Assignment  IndexMode=Zero-based  SampleTime=TimeStep  IndexOptions=Starting index (dialog)  Indices=PortIndex  OutputSizes=[1 1]
  Data Store Read : DataStoreRead  DataStoreName=SimCoreActuators  SampleTime=TimeStep
  Data Store Write : DataStoreWrite  DataStoreName=SimCoreActuators
  wires:
  Assignment/1 -> Data Store Write/1
  Data Store Read/1 -> Assignment/1
  Y/1 -> Assignment/2

== system V2x_TC_CarBreakdownWarning_cs/STATE_CameraTrolley/velRPY ==
  Y : Inport
  Assignment : Assignment  IndexMode=Zero-based  SampleTime=TimeStep  IndexOptions=Starting index (dialog)  Indices=PortIndex  OutputSizes=[1 1]
  Data Store Read : DataStoreRead  DataStoreName=SimCoreActuators  SampleTime=TimeStep
  Data Store Write : DataStoreWrite  DataStoreName=SimCoreActuators
  wires:
  Assignment/1 -> Data Store Write/1
  Data Store Read/1 -> Assignment/1
  Y/1 -> Assignment/2

== system V2x_TC_CarBreakdownWarning_cs/STATE_Fiat_Bravo_1/Acceleration ==
  Y : Inport
  Assignment : Assignment  IndexMode=Zero-based  SampleTime=TimeStep  IndexOptions=Starting index (dialog)  Indices=PortIndex  OutputSizes=[1 1]
  Data Store Read : DataStoreRead  DataStoreName=SimCoreActuators  SampleTime=TimeStep
  Data Store Write : DataStoreWrite  DataStoreName=SimCoreActuators
  wires:
  Assignment/1 -> Data Store Write/1
  Data Store Read/1 -> Assignment/1
  Y/1 -> Assignment/2

== system V2x_TC_CarBreakdownWarning_cs/STATE_Fiat_Bravo_1/Position ==
  Y : Inport
  Assignment : Assignment  IndexMode=Zero-based  SampleTime=TimeStep  IndexOptions=Starting index (dialog)  Indices=PortIndex  OutputSizes=[1 1]
  Data Store Read : DataStoreRead  DataStoreName=SimCoreActuators  SampleTime=TimeStep
  Data Store Write : DataStoreWrite  DataStoreName=SimCoreActuators
  wires:
  Y/1 -> Assignment/2
  Data Store Read/1 -> Assignment/1
  Assignment/1 -> Data Store Write/1

== system V2x_TC_CarBreakdownWarning_cs/STATE_Fiat_Bravo_1/RPY ==
  Y : Inport
  Assignment : Assignment  IndexMode=Zero-based  SampleTime=TimeStep  IndexOptions=Starting index (dialog)  Indices=PortIndex  OutputSizes=[1 1]
  Data Store Read : DataStoreRead  DataStoreName=SimCoreActuators  SampleTime=TimeStep
  Data Store Write : DataStoreWrite  DataStoreName=SimCoreActuators
  wires:
  Assignment/1 -> Data Store Write/1
  Data Store Read/1 -> Assignment/1
  Y/1 -> Assignment/2

== system V2x_TC_CarBreakdownWarning_cs/STATE_Fiat_Bravo_1/Velocity ==
  Y : Inport
  Assignment : Assignment  IndexMode=Zero-based  SampleTime=TimeStep  IndexOptions=Starting index (dialog)  Indices=PortIndex  OutputSizes=[1 1]
  Data Store Read : DataStoreRead  DataStoreName=SimCoreActuators  SampleTime=TimeStep
  Data Store Write : DataStoreWrite  DataStoreName=SimCoreActuators
  wires:
  Assignment/1 -> Data Store Write/1
  Data Store Read/1 -> Assignment/1
  Y/1 -> Assignment/2

== system V2x_TC_CarBreakdownWarning_cs/STATE_Fiat_Bravo_1/velRPY ==
  Y : Inport
  Assignment : Assignment  IndexMode=Zero-based  SampleTime=TimeStep  IndexOptions=Starting index (dialog)  Indices=PortIndex  OutputSizes=[1 1]
  Data Store Read : DataStoreRead  DataStoreName=SimCoreActuators  SampleTime=TimeStep
  Data Store Write : DataStoreWrite  DataStoreName=SimCoreActuators
  wires:
  Assignment/1 -> Data Store Write/1
  Data Store Read/1 -> Assignment/1
  Y/1 -> Assignment/2

== system V2x_TC_CarBreakdownWarning_cs/STATE_Toyota_Previa_1/Acceleration ==
  Y : Inport
  Assignment : Assignment  IndexMode=Zero-based  SampleTime=TimeStep  IndexOptions=Starting index (dialog)  Indices=PortIndex  OutputSizes=[1 1]
  Data Store Read : DataStoreRead  DataStoreName=SimCoreActuators  SampleTime=TimeStep
  Data Store Write : DataStoreWrite  DataStoreName=SimCoreActuators
  wires:
  Assignment/1 -> Data Store Write/1
  Data Store Read/1 -> Assignment/1
  Y/1 -> Assignment/2

== system V2x_TC_CarBreakdownWarning_cs/STATE_Toyota_Previa_1/Position ==
  Y : Inport
  Assignment : Assignment  IndexMode=Zero-based  SampleTime=TimeStep  IndexOptions=Starting index (dialog)  Indices=PortIndex  OutputSizes=[1 1]
  Data Store Read : DataStoreRead  DataStoreName=SimCoreActuators  SampleTime=TimeStep
  Data Store Write : DataStoreWrite  DataStoreName=SimCoreActuators
  wires:
  Y/1 -> Assignment/2
  Data Store Read/1 -> Assignment/1
  Assignment/1 -> Data Store Write/1

== system V2x_TC_CarBreakdownWarning_cs/STATE_Toyota_Previa_1/RPY ==
  Y : Inport
  Assignment : Assignment  IndexMode=Zero-based  SampleTime=TimeStep  IndexOptions=Starting index (dialog)  Indices=PortIndex  OutputSizes=[1 1]
  Data Store Read : DataStoreRead  DataStoreName=SimCoreActuators  SampleTime=TimeStep
  Data Store Write : DataStoreWrite  DataStoreName=SimCoreActuators
  wires:
  Assignment/1 -> Data Store Write/1
  Data Store Read/1 -> Assignment/1
  Y/1 -> Assignment/2

== system V2x_TC_CarBreakdownWarning_cs/STATE_Toyota_Previa_1/Velocity ==
  Y : Inport
  Assignment : Assignment  IndexMode=Zero-based  SampleTime=TimeStep  IndexOptions=Starting index (dialog)  Indices=PortIndex  OutputSizes=[1 1]
  Data Store Read : DataStoreRead  DataStoreName=SimCoreActuators  SampleTime=TimeStep
  Data Store Write : DataStoreWrite  DataStoreName=SimCoreActuators
  wires:
  Assignment/1 -> Data Store Write/1
  Data Store Read/1 -> Assignment/1
  Y/1 -> Assignment/2

== system V2x_TC_CarBreakdownWarning_cs/STATE_Toyota_Previa_1/velRPY ==
  Y : Inport
  Assignment : Assignment  IndexMode=Zero-based  SampleTime=TimeStep  IndexOptions=Starting index (dialog)  Indices=PortIndex  OutputSizes=[1 1]
  Data Store Read : DataStoreRead  DataStoreName=SimCoreActuators  SampleTime=TimeStep
  Data Store Write : DataStoreWrite  DataStoreName=SimCoreActuators
  wires:
  Assignment/1 -> Data Store Write/1
  Data Store Read/1 -> Assignment/1
  Y/1 -> Assignment/2
